simulink model "v2x_cs"  (R2019a)
settings: Solver=ode5  StartTime=0.0  StopTime=inf  FixedStep=1/20  RelTol=1e-3
PreLoadFcn:
  | mbxruntime.callbacks.PreLoadFcn(bdroot);
PostLoadFcn:
  | mbxruntime.callbacks.PostLoadFcn(bdroot);
InitFcn:
  | mbxruntime.callbacks.InitFcn(bdroot);
StartFcn:
  | mbxruntime.callbacks.StartFcn(bdroot);
StopFcn:
  | mbxruntime.callbacks.StopFcn(bdroot);
model workspace (MAT data in the model file):
  mbox_table : struct (value not decoded)
  model_closed = 0
  sim_status = 0
undefined symbols (not defined in the file or in its folder): DiscIntNeverNeededParam, SteeringWheel
libraries: PreScanSimulinkLibrary x10
(part 4 of 5)

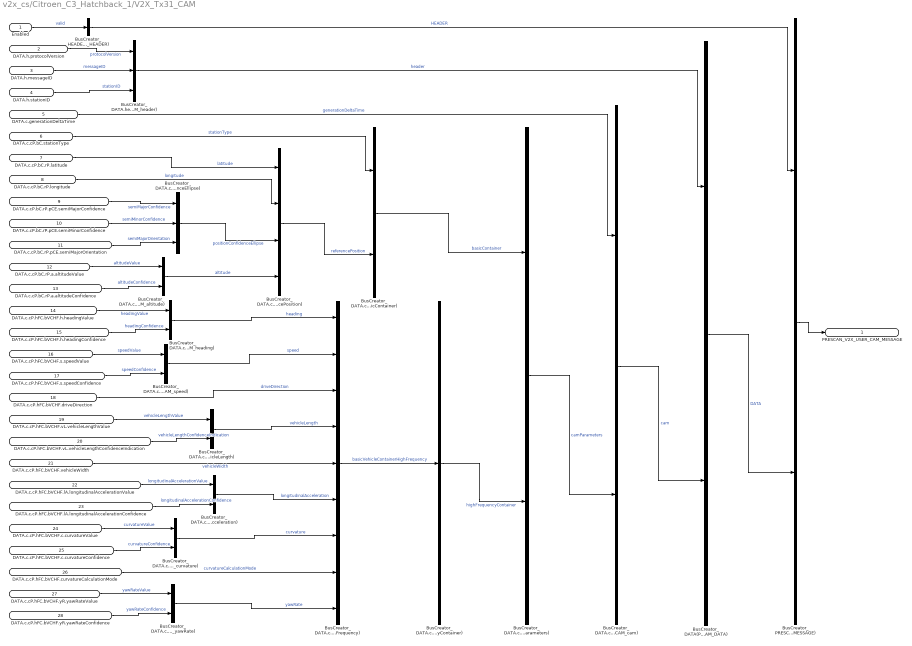
== system v2x_cs/Citroen_C3_Hatchback_1/V2X_Tx31_CAM ==
  Enabled : Inport
  DATA.h.protocolVersion : Inport  Port=2
  DATA.h.messageID : Inport  Port=3
  DATA.h.stationID : Inport  Port=4
  DATA.c.generationDeltaTime : Inport  Port=5
  DATA.c.cP.bC.stationType : Inport  Port=6
  DATA.c.cP.bC.rP.latitude : Inport  Port=7
  DATA.c.cP.bC.rP.longitude : Inport  Port=8
  DATA.c.cP.bC.rP.pCE.semiMajorConfidence : Inport  Port=9
  DATA.c.cP.bC.rP.pCE.semiMinorConfidence : Inport  Port=10
  DATA.c.cP.bC.rP.pCE.semiMajorOrientation : Inport  Port=11
  DATA.c.cP.bC.rP.a.altitudeValue : Inport  Port=12
  DATA.c.cP.bC.rP.a.altitudeConfidence : Inport  Port=13
  DATA.c.cP.hFC.bVCHF.h.headingValue : Inport  Port=14
  DATA.c.cP.hFC.bVCHF.h.headingConfidence : Inport  Port=15
  DATA.c.cP.hFC.bVCHF.s.speedValue : Inport  Port=16
  DATA.c.cP.hFC.bVCHF.s.speedConfidence : Inport  Port=17
  DATA.c.cP.hFC.bVCHF.driveDirection : Inport  Port=18
  DATA.c.cP.hFC.bVCHF.vL.vehicleLengthValue : Inport  Port=19
  DATA.c.cP.hFC.bVCHF.vL.vehicleLengthConfidenceIndication : Inport  Port=20
  DATA.c.cP.hFC.bVCHF.vehicleWidth : Inport  Port=21
  DATA.c.cP.hFC.bVCHF.lA.longitudinalAccelerationValue : Inport  Port=22
  DATA.c.cP.hFC.bVCHF.lA.longitudinalAccelerationConfidence : Inport  Port=23
  DATA.c.cP.hFC.bVCHF.c.curvatureValue : Inport  Port=24
  DATA.c.cP.hFC.bVCHF.c.curvatureConfidence : Inport  Port=25
  DATA.c.cP.hFC.bVCHF.curvatureCalculationMode : Inport  Port=26
  DATA.c.cP.hFC.bVCHF.yR.yawRateValue : Inport  Port=27
  DATA.c.cP.hFC.bVCHF.yR.yawRateConfidence : Inport  Port=28
  BusCreator_DATA(PRESCAN_V2X_USER_CAM_DATA) : BusCreator  Inputs=2  OutDataTypeStr=Bus: PRESCAN_V2X_USER_CAM_DATA  NonVirtualBus=on
  BusCreator_DATA.c.cP.bC.rP.altitude(PRESCAN_V2X_USER_CAM_altitude) : BusCreator  Inputs=2  OutDataTypeStr=Bus: PRESCAN_V2X_USER_CAM_altitude  NonVirtualBus=on
  BusCreator_DATA.c.cP.bC.rP.positionConfidenceEllipse(PRESCAN_V2X_USER_CAM_positionConfidenceEllipse) : BusCreator  Inputs=3  OutDataTypeStr=Bus: PRESCAN_V2X_USER_CAM_positionConfidenceEllipse  NonVirtualBus=on
  BusCreator_DATA.c.cP.bC.referencePosition(PRESCAN_V2X_USER_CAM_referencePosition) : BusCreator  Inputs=4  OutDataTypeStr=Bus: PRESCAN_V2X_USER_CAM_referencePosition  NonVirtualBus=on
  BusCreator_DATA.c.cP.basicContainer(PRESCAN_V2X_USER_CAM_basicContainer) : BusCreator  Inputs=2  OutDataTypeStr=Bus: PRESCAN_V2X_USER_CAM_basicContainer  NonVirtualBus=on
  BusCreator_DATA.c.cP.hFC.bVCHF.curvature(PRESCAN_V2X_USER_CAM_curvature) : BusCreator  Inputs=2  OutDataTypeStr=Bus: PRESCAN_V2X_USER_CAM_curvature  NonVirtualBus=on
  BusCreator_DATA.c.cP.hFC.bVCHF.heading(PRESCAN_V2X_USER_CAM_heading) : BusCreator  Inputs=2  OutDataTypeStr=Bus: PRESCAN_V2X_USER_CAM_heading  NonVirtualBus=on
  BusCreator_DATA.c.cP.hFC.bVCHF.longitudinalAcceleration(PRESCAN_V2X_USER_CAM_longitudinalAcceleration) : BusCreator  Inputs=2  OutDataTypeStr=Bus: PRESCAN_V2X_USER_CAM_longitudinalAcceleration  NonVirtualBus=on
  BusCreator_DATA.c.cP.hFC.bVCHF.speed(PRESCAN_V2X_USER_CAM_speed) : BusCreator  Inputs=2  OutDataTypeStr=Bus: PRESCAN_V2X_USER_CAM_speed  NonVirtualBus=on
  BusCreator_DATA.c.cP.hFC.bVCHF.vehicleLength(PRESCAN_V2X_USER_CAM_vehicleLength) : BusCreator  Inputs=2  OutDataTypeStr=Bus: PRESCAN_V2X_USER_CAM_vehicleLength  NonVirtualBus=on
  BusCreator_DATA.c.cP.hFC.bVCHF.yawRate(PRESCAN_V2X_USER_CAM_yawRate) : BusCreator  Inputs=2  OutDataTypeStr=Bus: PRESCAN_V2X_USER_CAM_yawRate  NonVirtualBus=on
  BusCreator_DATA.c.cP.hFC.basicVehicleContainerHighFrequency(PRESCAN_V2X_USER_CAM_basicVehicleContainerHighFrequency) : BusCreator  Inputs=9  OutDataTypeStr=Bus: PRESCAN_V2X_USER_CAM_basicVehicleContainerHighFrequency  NonVirtualBus=on
  BusCreator_DATA.c.cP.highFrequencyContainer(PRESCAN_V2X_USER_CAM_highFrequencyContainer) : BusCreator  Inputs=1  OutDataTypeStr=Bus: PRESCAN_V2X_USER_CAM_highFrequencyContainer  NonVirtualBus=on
  BusCreator_DATA.c.camParameters(PRESCAN_V2X_USER_CAM_camParameters) : BusCreator  Inputs=2  OutDataTypeStr=Bus: PRESCAN_V2X_USER_CAM_camParameters  NonVirtualBus=on
  BusCreator_DATA.cam(PRESCAN_V2X_USER_CAM_cam) : BusCreator  Inputs=2  OutDataTypeStr=Bus: PRESCAN_V2X_USER_CAM_cam  NonVirtualBus=on
  BusCreator_DATA.header(PRESCAN_V2X_USER_CAM_header) : BusCreator  Inputs=3  OutDataTypeStr=Bus: PRESCAN_V2X_USER_CAM_header  NonVirtualBus=on
  BusCreator_HEADER(PRESCAN_HEADER) : BusCreator  Inputs=1  OutDataTypeStr=Bus: PRESCAN_HEADER  NonVirtualBus=on
  BusCreator_PRESCAN_V2X_USER_CAM_MESSAGE(PRESCAN_V2X_USER_CAM_MESSAGE) : BusCreator  Inputs=2  OutDataTypeStr=Bus: PRESCAN_V2X_USER_CAM_MESSAGE  NonVirtualBus=on
  PRESCAN_V2X_USER_CAM_MESSAGE : Outport
  wires:
  Enabled/1 -> BusCreator_HEADER(PRESCAN_HEADER)/1  "valid"
  DATA.h.messageID/1 -> BusCreator_DATA.header(PRESCAN_V2X_USER_CAM_header)/2  "messageID"
  DATA.h.stationID/1 -> BusCreator_DATA.header(PRESCAN_V2X_USER_CAM_header)/3  "stationID"
  DATA.h.protocolVersion/1 -> BusCreator_DATA.header(PRESCAN_V2X_USER_CAM_header)/1  "protocolVersion"
  DATA.c.cP.bC.rP.pCE.semiMinorConfidence/1 -> BusCreator_DATA.c.cP.bC.rP.positionConfidenceEllipse(PRESCAN_V2X_USER_CAM_positionConfidenceEllipse)/2  "semiMinorConfidence"
  DATA.c.cP.bC.rP.pCE.semiMajorOrientation/1 -> BusCreator_DATA.c.cP.bC.rP.positionConfidenceEllipse(PRESCAN_V2X_USER_CAM_positionConfidenceEllipse)/3  "semiMajorOrientation"
  DATA.c.cP.bC.rP.pCE.semiMajorConfidence/1 -> BusCreator_DATA.c.cP.bC.rP.positionConfidenceEllipse(PRESCAN_V2X_USER_CAM_positionConfidenceEllipse)/1  "semiMajorConfidence"
  DATA.c.cP.bC.rP.a.altitudeValue/1 -> BusCreator_DATA.c.cP.bC.rP.altitude(PRESCAN_V2X_USER_CAM_altitude)/1  "altitudeValue"
  DATA.c.cP.bC.rP.a.altitudeConfidence/1 -> BusCreator_DATA.c.cP.bC.rP.altitude(PRESCAN_V2X_USER_CAM_altitude)/2  "altitudeConfidence"
  DATA.c.cP.bC.rP.longitude/1 -> BusCreator_DATA.c.cP.bC.referencePosition(PRESCAN_V2X_USER_CAM_referencePosition)/2  "longitude"
  BusCreator_DATA.c.cP.bC.rP.positionConfidenceEllipse(PRESCAN_V2X_USER_CAM_positionConfidenceEllipse)/1 -> BusCreator_DATA.c.cP.bC.referencePosition(PRESCAN_V2X_USER_CAM_referencePosition)/3  "positionConfidenceEllipse"
  DATA.c.cP.bC.rP.latitude/1 -> BusCreator_DATA.c.cP.bC.referencePosition(PRESCAN_V2X_USER_CAM_referencePosition)/1  "latitude"
  BusCreator_DATA.c.cP.bC.rP.altitude(PRESCAN_V2X_USER_CAM_altitude)/1 -> BusCreator_DATA.c.cP.bC.referencePosition(PRESCAN_V2X_USER_CAM_referencePosition)/4  "altitude"
  DATA.c.cP.bC.stationType/1 -> BusCreator_DATA.c.cP.basicContainer(PRESCAN_V2X_USER_CAM_basicContainer)/1  "stationType"
  BusCreator_DATA.c.cP.bC.referencePosition(PRESCAN_V2X_USER_CAM_referencePosition)/1 -> BusCreator_DATA.c.cP.basicContainer(PRESCAN_V2X_USER_CAM_basicContainer)/2  "referencePosition"
  DATA.c.cP.hFC.bVCHF.h.headingValue/1 -> BusCreator_DATA.c.cP.hFC.bVCHF.heading(PRESCAN_V2X_USER_CAM_heading)/1  "headingValue"
  DATA.c.cP.hFC.bVCHF.h.headingConfidence/1 -> BusCreator_DATA.c.cP.hFC.bVCHF.heading(PRESCAN_V2X_USER_CAM_heading)/2  "headingConfidence"
  DATA.c.cP.hFC.bVCHF.s.speedValue/1 -> BusCreator_DATA.c.cP.hFC.bVCHF.speed(PRESCAN_V2X_USER_CAM_speed)/1  "speedValue"
  DATA.c.cP.hFC.bVCHF.s.speedConfidence/1 -> BusCreator_DATA.c.cP.hFC.bVCHF.speed(PRESCAN_V2X_USER_CAM_speed)/2  "speedConfidence"
  DATA.c.cP.hFC.bVCHF.vL.vehicleLengthValue/1 -> BusCreator_DATA.c.cP.hFC.bVCHF.vehicleLength(PRESCAN_V2X_USER_CAM_vehicleLength)/1  "vehicleLengthValue"
  DATA.c.cP.hFC.bVCHF.vL.vehicleLengthConfidenceIndication/1 -> BusCreator_DATA.c.cP.hFC.bVCHF.vehicleLength(PRESCAN_V2X_USER_CAM_vehicleLength)/2  "vehicleLengthConfidenceIndication"
  DATA.c.cP.hFC.bVCHF.lA.longitudinalAccelerationValue/1 -> BusCreator_DATA.c.cP.hFC.bVCHF.longitudinalAcceleration(PRESCAN_V2X_USER_CAM_longitudinalAcceleration)/1  "longitudinalAccelerationValue"
  DATA.c.cP.hFC.bVCHF.lA.longitudinalAccelerationConfidence/1 -> BusCreator_DATA.c.cP.hFC.bVCHF.longitudinalAcceleration(PRESCAN_V2X_USER_CAM_longitudinalAcceleration)/2  "longitudinalAccelerationConfidence"
  DATA.c.cP.hFC.bVCHF.c.curvatureValue/1 -> BusCreator_DATA.c.cP.hFC.bVCHF.curvature(PRESCAN_V2X_USER_CAM_curvature)/1  "curvatureValue"
  DATA.c.cP.hFC.bVCHF.c.curvatureConfidence/1 -> BusCreator_DATA.c.cP.hFC.bVCHF.curvature(PRESCAN_V2X_USER_CAM_curvature)/2  "curvatureConfidence"
  DATA.c.cP.hFC.bVCHF.yR.yawRateValue/1 -> BusCreator_DATA.c.cP.hFC.bVCHF.yawRate(PRESCAN_V2X_USER_CAM_yawRate)/1  "yawRateValue"
  DATA.c.cP.hFC.bVCHF.yR.yawRateConfidence/1 -> BusCreator_DATA.c.cP.hFC.bVCHF.yawRate(PRESCAN_V2X_USER_CAM_yawRate)/2  "yawRateConfidence"
  DATA.c.cP.hFC.bVCHF.vehicleWidth/1 -> BusCreator_DATA.c.cP.hFC.basicVehicleContainerHighFrequency(PRESCAN_V2X_USER_CAM_basicVehicleContainerHighFrequency)/5  "vehicleWidth"
  BusCreator_DATA.c.cP.hFC.bVCHF.longitudinalAcceleration(PRESCAN_V2X_USER_CAM_longitudinalAcceleration)/1 -> BusCreator_DATA.c.cP.hFC.basicVehicleContainerHighFrequency(PRESCAN_V2X_USER_CAM_basicVehicleContainerHighFrequency)/6  "longitudinalAcceleration"
  BusCreator_DATA.c.cP.hFC.bVCHF.vehicleLength(PRESCAN_V2X_USER_CAM_vehicleLength)/1 -> BusCreator_DATA.c.cP.hFC.basicVehicleContainerHighFrequency(PRESCAN_V2X_USER_CAM_basicVehicleContainerHighFrequency)/4  "vehicleLength"
  BusCreator_DATA.c.cP.hFC.bVCHF.curvature(PRESCAN_V2X_USER_CAM_curvature)/1 -> BusCreator_DATA.c.cP.hFC.basicVehicleContainerHighFrequency(PRESCAN_V2X_USER_CAM_basicVehicleContainerHighFrequency)/7  "curvature"
  DATA.c.cP.hFC.bVCHF.driveDirection/1 -> BusCreator_DATA.c.cP.hFC.basicVehicleContainerHighFrequency(PRESCAN_V2X_USER_CAM_basicVehicleContainerHighFrequency)/3  "driveDirection"
  DATA.c.cP.hFC.bVCHF.curvatureCalculationMode/1 -> BusCreator_DATA.c.cP.hFC.basicVehicleContainerHighFrequency(PRESCAN_V2X_USER_CAM_basicVehicleContainerHighFrequency)/8  "curvatureCalculationMode"
  BusCreator_DATA.c.cP.hFC.bVCHF.speed(PRESCAN_V2X_USER_CAM_speed)/1 -> BusCreator_DATA.c.cP.hFC.basicVehicleContainerHighFrequency(PRESCAN_V2X_USER_CAM_basicVehicleContainerHighFrequency)/2  "speed"
  BusCreator_DATA.c.cP.hFC.bVCHF.yawRate(PRESCAN_V2X_USER_CAM_yawRate)/1 -> BusCreator_DATA.c.cP.hFC.basicVehicleContainerHighFrequency(PRESCAN_V2X_USER_CAM_basicVehicleContainerHighFrequency)/9  "yawRate"
  BusCreator_DATA.c.cP.hFC.bVCHF.heading(PRESCAN_V2X_USER_CAM_heading)/1 -> BusCreator_DATA.c.cP.hFC.basicVehicleContainerHighFrequency(PRESCAN_V2X_USER_CAM_basicVehicleContainerHighFrequency)/1  "heading"
  BusCreator_DATA.c.cP.hFC.basicVehicleContainerHighFrequency(PRESCAN_V2X_USER_CAM_basicVehicleContainerHighFrequency)/1 -> BusCreator_DATA.c.cP.highFrequencyContainer(PRESCAN_V2X_USER_CAM_highFrequencyContainer)/1  "basicVehicleContainerHighFrequency"
  BusCreator_DATA.c.cP.basicContainer(PRESCAN_V2X_USER_CAM_basicContainer)/1 -> BusCreator_DATA.c.camParameters(PRESCAN_V2X_USER_CAM_camParameters)/1  "basicContainer"
  BusCreator_DATA.c.cP.highFrequencyContainer(PRESCAN_V2X_USER_CAM_highFrequencyContainer)/1 -> BusCreator_DATA.c.camParameters(PRESCAN_V2X_USER_CAM_camParameters)/2  "highFrequencyContainer"
  DATA.c.generationDeltaTime/1 -> BusCreator_DATA.cam(PRESCAN_V2X_USER_CAM_cam)/1  "generationDeltaTime"
  BusCreator_DATA.c.camParameters(PRESCAN_V2X_USER_CAM_camParameters)/1 -> BusCreator_DATA.cam(PRESCAN_V2X_USER_CAM_cam)/2  "camParameters"
  BusCreator_DATA.header(PRESCAN_V2X_USER_CAM_header)/1 -> BusCreator_DATA(PRESCAN_V2X_USER_CAM_DATA)/1  "header"
  BusCreator_DATA.cam(PRESCAN_V2X_USER_CAM_cam)/1 -> BusCreator_DATA(PRESCAN_V2X_USER_CAM_DATA)/2  "cam"
  BusCreator_HEADER(PRESCAN_HEADER)/1 -> BusCreator_PRESCAN_V2X_USER_CAM_MESSAGE(PRESCAN_V2X_USER_CAM_MESSAGE)/1  "HEADER"
  BusCreator_DATA(PRESCAN_V2X_USER_CAM_DATA)/1 -> BusCreator_PRESCAN_V2X_USER_CAM_MESSAGE(PRESCAN_V2X_USER_CAM_MESSAGE)/2  "DATA"
  BusCreator_PRESCAN_V2X_USER_CAM_MESSAGE(PRESCAN_V2X_USER_CAM_MESSAGE)/1 -> PRESCAN_V2X_USER_CAM_MESSAGE/1

== system v2x_cs/Mazda_RX8_Coupe_1/Dynamics_Empty ==
  note: For state mode 'Dynamic' positions
      | are not taken into account, as they
      | are computed by integrating velocity.
      | Click annotation for Help.
  Ground_{1..9} (9 alike) : Ground
  MuxState : Subsystem  Tag=mux/State  mask(Empty Dynamics State Block){positioningmode=on, TimeStep=1/20}
      mask prompts: positioningmode "Positioning Mode"; TimeStep "Auto Assigned: Time Step [s]"
      mask help:
      | Build the state of an actor based on user input.
      | The user can either use positioning mode or dynamics mode.
      | - When using positioning mode the position and orientation of the actor are set directly based on the input. Expected input is relative to the initial position and orientation of the actor. It's also possible to specify the velocity of the actor, though this input isn't used, only passed on.
      | - When using dynamics mode the position input is ignored. Expected input is velocity and orientation. The velocity is relative the current orientation of the actor, while orientation is relative to its initial orientation. The position of the actor is calculated based on the velocity and orientation given.
      settings: DeleteFcn=PreScanBlockDeleteFcn;
  State : Outport  Tag=outport/StateOutport  SampleTime=1/20
  wires:
  MuxState/1(state) -> State/1
  Ground_1/1 -> MuxState/1(x [m])
  Ground_2/1 -> MuxState/2(y [m])
  Ground_3/1 -> MuxState/3(z [m])
  Ground_4/1 -> MuxState/4(dx [m/s])
  Ground_5/1 -> MuxState/5(dy [m/s])
  Ground_6/1 -> MuxState/6(dz [m/s])
  Ground_7/1 -> MuxState/7(R [rad])
  Ground_8/1 -> MuxState/8(P [rad])
  Ground_9/1 -> MuxState/9(Y [rad])

== system v2x_cs/Mazda_RX8_Coupe_1/SELF_Demux ==
  SELF : Inport  OutDataTypeStr=Bus: PRESCAN_SELFSENSORDATA
  Bus Selector : BusSelector  OutputSignals=PositionX,PositionY,PositionZ,OrientationRoll,OrientationPitch,OrientationYaw,Velocity,Yaw_rate,Lat,Long,Alt
  Demux2 : Demux  Outputs=3
  Gain : Gain  Gain=180/pi
  Gain1 : Gain  Gain=180/pi
  Vector Concatenate1 : Concatenate  NumInputs=3
  compas converter : Subsystem
  x [m] : Outport
  y [m] : Outport  Port=2
  z [m] : Outport  Port=3
  rotx [deg] : Outport  Port=4
  roty [deg] : Outport  Port=5
  rotz [deg] : Outport  Port=6
  GPS lat [deg] : Outport  Port=7
  GPS long [deg] : Outport  Port=8
  GPS alt [m] : Outport  Port=9
  velocity [m/s] : Outport  Port=10
  heading [deg] : Outport  Port=11
  yaw rate [deg/s] : Outport  Port=12
  wires:
  Bus Selector/11 -> GPS alt [m]/1  "<Alt>"
  Bus Selector/10 -> GPS long [deg]/1  "<Long>"
  Bus Selector/9 -> GPS lat [deg]/1  "<Lat>"
  Bus Selector/8 -> Gain1/1  "<Yaw_rate>"
  Bus Selector/7 -> velocity [m/s]/1  "<Velocity>"
  Bus Selector/6 -> compas converter/1(rotz [rad]), Vector Concatenate1/3  "<OrientationYaw>"
  Bus Selector/5 -> Vector Concatenate1/2  "<OrientationPitch>"
  Bus Selector/4 -> Vector Concatenate1/1  "<OrientationRoll>"
  Vector Concatenate1/1 -> Gain/1
  Bus Selector/3 -> z [m]/1  "<PositionZ>"
  Bus Selector/2 -> y [m]/1  "<PositionY>"
  Bus Selector/1 -> x [m]/1  "<PositionX>"
  SELF/1 -> Bus Selector/1
  Gain/1 -> Demux2/1
  Demux2/1 -> rotx [deg]/1
  Demux2/2 -> roty [deg]/1
  Demux2/3 -> rotz [deg]/1
  compas converter/1(heading [deg]) -> heading [deg]/1
  Gain1/1 -> yaw rate [deg/s]/1

== system v2x_cs/Mazda_RX8_Coupe_1/STATE_Mazda_RX8_Coupe_1 ==
  State : Inport  SampleTime=TimeStep
  Bus Creator : BusCreator  Inputs=15  OutDataTypeStr=Bus: PRESCAN_STATEACTUATORDATA  NonVirtualBus=on
  Demux : Demux  Outputs=15
  iniBODYAngles wrtVEH [rad] : Constant  Value=[Roll0 Pitch0 0]  SampleTime=TimeStep
  iniVEHAngles wrtGLOB [rad] : Constant  Value=[0 0 Yaw0]  SampleTime=TimeStep
  iniVEHposition wrtGLOB [m] : Constant  Value=[x0 y0 z0]  SampleTime=TimeStep
  state2FullState : PreScanSimulinkLibrary/state2FullState  SystemSampleTime=-1
  StateBus : Outport  OutDataTypeStr=Bus: PRESCAN_STATEACTUATORDATA
  wires:
  Bus Creator/1 -> StateBus/1
  State/1 -> state2FullState/1
  state2FullState/1 -> Demux/1
  iniVEHposition wrtGLOB [m]/1 -> state2FullState/2
  iniBODYAngles wrtVEH [rad]/1 -> state2FullState/3
  iniVEHAngles wrtGLOB [rad]/1 -> state2FullState/4
  Demux/1 -> Bus Creator/1  "PositionX"
  Demux/2 -> Bus Creator/2  "PositionY"
  Demux/3 -> Bus Creator/3  "PositionZ"
  Demux/4 -> Bus Creator/4  "VelocityX"
  Demux/5 -> Bus Creator/5  "VelocityY"
  Demux/6 -> Bus Creator/6  "VelocityZ"
  Demux/7 -> Bus Creator/7  "AccelerationX"
  Demux/8 -> Bus Creator/8  "AccelerationY"
  Demux/9 -> Bus Creator/9  "AccelerationZ"
  Demux/10 -> Bus Creator/10  "OrientationRoll"
  Demux/11 -> Bus Creator/11  "OrientationPitch"
  Demux/12 -> Bus Creator/12  "OrientationYaw"
  Demux/13 -> Bus Creator/13  "AngularVelocityRoll"
  Demux/14 -> Bus Creator/14  "AngularVelocityPitch"
  Demux/15 -> Bus Creator/15  "AngularVelocityYaw"

== system v2x_cs/Mazda_RX8_Coupe_1/SteeringWheel_pivot_Mux ==
  X [m] : Inport
  Y [m] : Inport  Port=2
  Z [m] : Inport  Port=3
  Roll [rad] : Inport  Port=4
  Pitch [rad] : Inport  Port=5
  Yaw [rad] : Inport  Port=6
  Bus Creator : BusCreator  Inputs=3  OutDataTypeStr=Bus: PRESCAN_XYZ_DATA
  Bus Creator1 : BusCreator  Inputs=3  OutDataTypeStr=Bus: PRESCAN_RPY_DATA
  Bus Creator2 : BusCreator  Inputs=2  OutDataTypeStr=Bus: PRESCAN_POSE_DATA
  Joint : Outport
  wires:
  Yaw [rad]/1 -> Bus Creator1/3  "Yaw"
  Bus Creator1/1 -> Bus Creator2/2  "ORIENTATION"
  Bus Creator/1 -> Bus Creator2/1  "POSITION"
  X [m]/1 -> Bus Creator/1  "X"
  Y [m]/1 -> Bus Creator/2  "Y"
  Z [m]/1 -> Bus Creator/3  "Z"
  Bus Creator2/1 -> Joint/1
  Roll [rad]/1 -> Bus Creator1/1  "Roll"
  Pitch [rad]/1 -> Bus Creator1/2  "Pitch"

== system v2x_cs/Mazda_RX8_Coupe_1/V2X_27_CAM_Expander ==
  In : Inport
  Expander : MATLAB Function  TreatAsAtomicUnit=on
  Zero : Constant  Value=0  OutDataTypeStr=Bus: PRESCAN_V2X_FIXED_CAM_MESSAGE
  Out : Outport
  wires:
  In/1 -> Expander/1(u)
  Expander/1(y) -> Out/1
  Zero/1 -> Expander/2(z)

== system v2x_cs/Mazda_RX8_Coupe_1/V2X_27_CAM_Filter ==
  Filter_In : Inport  Partition=on  PartitionDimension=1  PartitionWidth=1  PartitionOffset=0
  Filter : Subsystem
  ForEach : ForEach
  Filter_Out : Outport  ConcatenationDimension=1
  wires:
  Filter_In/1 -> Filter/1(In)
  Filter/1(Out) -> Filter_Out/1

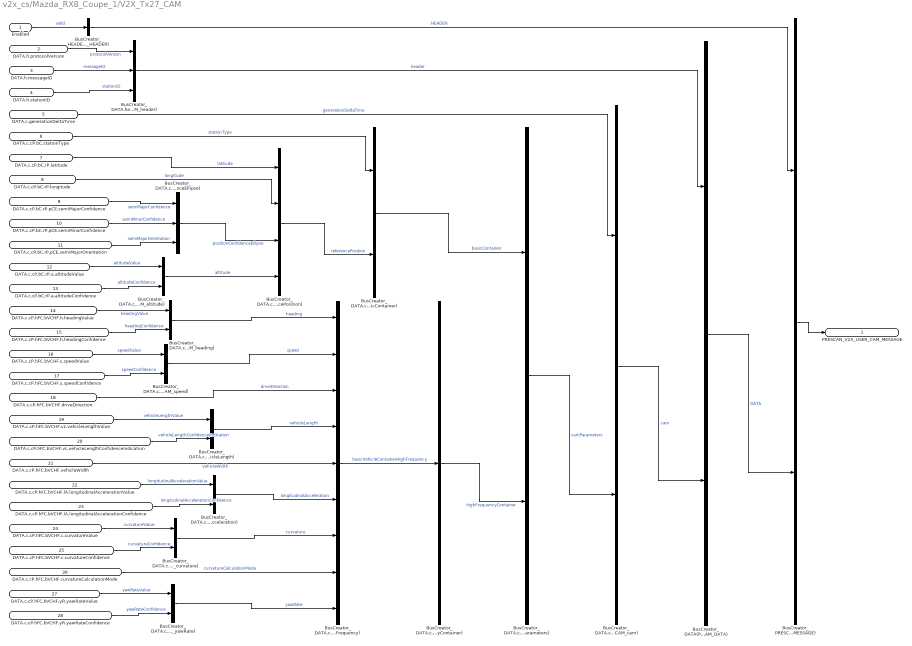
== system v2x_cs/Mazda_RX8_Coupe_1/V2X_Tx27_CAM ==
  Enabled : Inport
  DATA.h.protocolVersion : Inport  Port=2
  DATA.h.messageID : Inport  Port=3
  DATA.h.stationID : Inport  Port=4
  DATA.c.generationDeltaTime : Inport  Port=5
  DATA.c.cP.bC.stationType : Inport  Port=6
  DATA.c.cP.bC.rP.latitude : Inport  Port=7
  DATA.c.cP.bC.rP.longitude : Inport  Port=8
  DATA.c.cP.bC.rP.pCE.semiMajorConfidence : Inport  Port=9
  DATA.c.cP.bC.rP.pCE.semiMinorConfidence : Inport  Port=10
  DATA.c.cP.bC.rP.pCE.semiMajorOrientation : Inport  Port=11
  DATA.c.cP.bC.rP.a.altitudeValue : Inport  Port=12
  DATA.c.cP.bC.rP.a.altitudeConfidence : Inport  Port=13
  DATA.c.cP.hFC.bVCHF.h.headingValue : Inport  Port=14
  DATA.c.cP.hFC.bVCHF.h.headingConfidence : Inport  Port=15
  DATA.c.cP.hFC.bVCHF.s.speedValue : Inport  Port=16
  DATA.c.cP.hFC.bVCHF.s.speedConfidence : Inport  Port=17
  DATA.c.cP.hFC.bVCHF.driveDirection : Inport  Port=18
  DATA.c.cP.hFC.bVCHF.vL.vehicleLengthValue : Inport  Port=19
  DATA.c.cP.hFC.bVCHF.vL.vehicleLengthConfidenceIndication : Inport  Port=20
  DATA.c.cP.hFC.bVCHF.vehicleWidth : Inport  Port=21
  DATA.c.cP.hFC.bVCHF.lA.longitudinalAccelerationValue : Inport  Port=22
  DATA.c.cP.hFC.bVCHF.lA.longitudinalAccelerationConfidence : Inport  Port=23
  DATA.c.cP.hFC.bVCHF.c.curvatureValue : Inport  Port=24
  DATA.c.cP.hFC.bVCHF.c.curvatureConfidence : Inport  Port=25
  DATA.c.cP.hFC.bVCHF.curvatureCalculationMode : Inport  Port=26
  DATA.c.cP.hFC.bVCHF.yR.yawRateValue : Inport  Port=27
  DATA.c.cP.hFC.bVCHF.yR.yawRateConfidence : Inport  Port=28
  BusCreator_DATA(PRESCAN_V2X_USER_CAM_DATA) : BusCreator  Inputs=2  OutDataTypeStr=Bus: PRESCAN_V2X_USER_CAM_DATA  NonVirtualBus=on
  BusCreator_DATA.c.cP.bC.rP.altitude(PRESCAN_V2X_USER_CAM_altitude) : BusCreator  Inputs=2  OutDataTypeStr=Bus: PRESCAN_V2X_USER_CAM_altitude  NonVirtualBus=on
  BusCreator_DATA.c.cP.bC.rP.positionConfidenceEllipse(PRESCAN_V2X_USER_CAM_positionConfidenceEllipse) : BusCreator  Inputs=3  OutDataTypeStr=Bus: PRESCAN_V2X_USER_CAM_positionConfidenceEllipse  NonVirtualBus=on
  BusCreator_DATA.c.cP.bC.referencePosition(PRESCAN_V2X_USER_CAM_referencePosition) : BusCreator  Inputs=4  OutDataTypeStr=Bus: PRESCAN_V2X_USER_CAM_referencePosition  NonVirtualBus=on
  BusCreator_DATA.c.cP.basicContainer(PRESCAN_V2X_USER_CAM_basicContainer) : BusCreator  Inputs=2  OutDataTypeStr=Bus: PRESCAN_V2X_USER_CAM_basicContainer  NonVirtualBus=on
  BusCreator_DATA.c.cP.hFC.bVCHF.curvature(PRESCAN_V2X_USER_CAM_curvature) : BusCreator  Inputs=2  OutDataTypeStr=Bus: PRESCAN_V2X_USER_CAM_curvature  NonVirtualBus=on
  BusCreator_DATA.c.cP.hFC.bVCHF.heading(PRESCAN_V2X_USER_CAM_heading) : BusCreator  Inputs=2  OutDataTypeStr=Bus: PRESCAN_V2X_USER_CAM_heading  NonVirtualBus=on
  BusCreator_DATA.c.cP.hFC.bVCHF.longitudinalAcceleration(PRESCAN_V2X_USER_CAM_longitudinalAcceleration) : BusCreator  Inputs=2  OutDataTypeStr=Bus: PRESCAN_V2X_USER_CAM_longitudinalAcceleration  NonVirtualBus=on
  BusCreator_DATA.c.cP.hFC.bVCHF.speed(PRESCAN_V2X_USER_CAM_speed) : BusCreator  Inputs=2  OutDataTypeStr=Bus: PRESCAN_V2X_USER_CAM_speed  NonVirtualBus=on
  BusCreator_DATA.c.cP.hFC.bVCHF.vehicleLength(PRESCAN_V2X_USER_CAM_vehicleLength) : BusCreator  Inputs=2  OutDataTypeStr=Bus: PRESCAN_V2X_USER_CAM_vehicleLength  NonVirtualBus=on
  BusCreator_DATA.c.cP.hFC.bVCHF.yawRate(PRESCAN_V2X_USER_CAM_yawRate) : BusCreator  Inputs=2  OutDataTypeStr=Bus: PRESCAN_V2X_USER_CAM_yawRate  NonVirtualBus=on
  BusCreator_DATA.c.cP.hFC.basicVehicleContainerHighFrequency(PRESCAN_V2X_USER_CAM_basicVehicleContainerHighFrequency) : BusCreator  Inputs=9  OutDataTypeStr=Bus: PRESCAN_V2X_USER_CAM_basicVehicleContainerHighFrequency  NonVirtualBus=on
  BusCreator_DATA.c.cP.highFrequencyContainer(PRESCAN_V2X_USER_CAM_highFrequencyContainer) : BusCreator  Inputs=1  OutDataTypeStr=Bus: PRESCAN_V2X_USER_CAM_highFrequencyContainer  NonVirtualBus=on
  BusCreator_DATA.c.camParameters(PRESCAN_V2X_USER_CAM_camParameters) : BusCreator  Inputs=2  OutDataTypeStr=Bus: PRESCAN_V2X_USER_CAM_camParameters  NonVirtualBus=on
  BusCreator_DATA.cam(PRESCAN_V2X_USER_CAM_cam) : BusCreator  Inputs=2  OutDataTypeStr=Bus: PRESCAN_V2X_USER_CAM_cam  NonVirtualBus=on
  BusCreator_DATA.header(PRESCAN_V2X_USER_CAM_header) : BusCreator  Inputs=3  OutDataTypeStr=Bus: PRESCAN_V2X_USER_CAM_header  NonVirtualBus=on
  BusCreator_HEADER(PRESCAN_HEADER) : BusCreator  Inputs=1  OutDataTypeStr=Bus: PRESCAN_HEADER  NonVirtualBus=on
  BusCreator_PRESCAN_V2X_USER_CAM_MESSAGE(PRESCAN_V2X_USER_CAM_MESSAGE) : BusCreator  Inputs=2  OutDataTypeStr=Bus: PRESCAN_V2X_USER_CAM_MESSAGE  NonVirtualBus=on
  PRESCAN_V2X_USER_CAM_MESSAGE : Outport
  wires:
  Enabled/1 -> BusCreator_HEADER(PRESCAN_HEADER)/1  "valid"
  DATA.h.messageID/1 -> BusCreator_DATA.header(PRESCAN_V2X_USER_CAM_header)/2  "messageID"
  DATA.h.stationID/1 -> BusCreator_DATA.header(PRESCAN_V2X_USER_CAM_header)/3  "stationID"
  DATA.h.protocolVersion/1 -> BusCreator_DATA.header(PRESCAN_V2X_USER_CAM_header)/1  "protocolVersion"
  DATA.c.cP.bC.rP.pCE.semiMinorConfidence/1 -> BusCreator_DATA.c.cP.bC.rP.positionConfidenceEllipse(PRESCAN_V2X_USER_CAM_positionConfidenceEllipse)/2  "semiMinorConfidence"
  DATA.c.cP.bC.rP.pCE.semiMajorOrientation/1 -> BusCreator_DATA.c.cP.bC.rP.positionConfidenceEllipse(PRESCAN_V2X_USER_CAM_positionConfidenceEllipse)/3  "semiMajorOrientation"
  DATA.c.cP.bC.rP.pCE.semiMajorConfidence/1 -> BusCreator_DATA.c.cP.bC.rP.positionConfidenceEllipse(PRESCAN_V2X_USER_CAM_positionConfidenceEllipse)/1  "semiMajorConfidence"
  DATA.c.cP.bC.rP.a.altitudeValue/1 -> BusCreator_DATA.c.cP.bC.rP.altitude(PRESCAN_V2X_USER_CAM_altitude)/1  "altitudeValue"
  DATA.c.cP.bC.rP.a.altitudeConfidence/1 -> BusCreator_DATA.c.cP.bC.rP.altitude(PRESCAN_V2X_USER_CAM_altitude)/2  "altitudeConfidence"
  DATA.c.cP.bC.rP.longitude/1 -> BusCreator_DATA.c.cP.bC.referencePosition(PRESCAN_V2X_USER_CAM_referencePosition)/2  "longitude"
  BusCreator_DATA.c.cP.bC.rP.positionConfidenceEllipse(PRESCAN_V2X_USER_CAM_positionConfidenceEllipse)/1 -> BusCreator_DATA.c.cP.bC.referencePosition(PRESCAN_V2X_USER_CAM_referencePosition)/3  "positionConfidenceEllipse"
  DATA.c.cP.bC.rP.latitude/1 -> BusCreator_DATA.c.cP.bC.referencePosition(PRESCAN_V2X_USER_CAM_referencePosition)/1  "latitude"
  BusCreator_DATA.c.cP.bC.rP.altitude(PRESCAN_V2X_USER_CAM_altitude)/1 -> BusCreator_DATA.c.cP.bC.referencePosition(PRESCAN_V2X_USER_CAM_referencePosition)/4  "altitude"
  DATA.c.cP.bC.stationType/1 -> BusCreator_DATA.c.cP.basicContainer(PRESCAN_V2X_USER_CAM_basicContainer)/1  "stationType"
  BusCreator_DATA.c.cP.bC.referencePosition(PRESCAN_V2X_USER_CAM_referencePosition)/1 -> BusCreator_DATA.c.cP.basicContainer(PRESCAN_V2X_USER_CAM_basicContainer)/2  "referencePosition"
  DATA.c.cP.hFC.bVCHF.h.headingValue/1 -> BusCreator_DATA.c.cP.hFC.bVCHF.heading(PRESCAN_V2X_USER_CAM_heading)/1  "headingValue"
  DATA.c.cP.hFC.bVCHF.h.headingConfidence/1 -> BusCreator_DATA.c.cP.hFC.bVCHF.heading(PRESCAN_V2X_USER_CAM_heading)/2  "headingConfidence"
  DATA.c.cP.hFC.bVCHF.s.speedValue/1 -> BusCreator_DATA.c.cP.hFC.bVCHF.speed(PRESCAN_V2X_USER_CAM_speed)/1  "speedValue"
  DATA.c.cP.hFC.bVCHF.s.speedConfidence/1 -> BusCreator_DATA.c.cP.hFC.bVCHF.speed(PRESCAN_V2X_USER_CAM_speed)/2  "speedConfidence"
  DATA.c.cP.hFC.bVCHF.vL.vehicleLengthValue/1 -> BusCreator_DATA.c.cP.hFC.bVCHF.vehicleLength(PRESCAN_V2X_USER_CAM_vehicleLength)/1  "vehicleLengthValue"
  DATA.c.cP.hFC.bVCHF.vL.vehicleLengthConfidenceIndication/1 -> BusCreator_DATA.c.cP.hFC.bVCHF.vehicleLength(PRESCAN_V2X_USER_CAM_vehicleLength)/2  "vehicleLengthConfidenceIndication"
  DATA.c.cP.hFC.bVCHF.lA.longitudinalAccelerationValue/1 -> BusCreator_DATA.c.cP.hFC.bVCHF.longitudinalAcceleration(PRESCAN_V2X_USER_CAM_longitudinalAcceleration)/1  "longitudinalAccelerationValue"
  DATA.c.cP.hFC.bVCHF.lA.longitudinalAccelerationConfidence/1 -> BusCreator_DATA.c.cP.hFC.bVCHF.longitudinalAcceleration(PRESCAN_V2X_USER_CAM_longitudinalAcceleration)/2  "longitudinalAccelerationConfidence"
  DATA.c.cP.hFC.bVCHF.c.curvatureValue/1 -> BusCreator_DATA.c.cP.hFC.bVCHF.curvature(PRESCAN_V2X_USER_CAM_curvature)/1  "curvatureValue"
  DATA.c.cP.hFC.bVCHF.c.curvatureConfidence/1 -> BusCreator_DATA.c.cP.hFC.bVCHF.curvature(PRESCAN_V2X_USER_CAM_curvature)/2  "curvatureConfidence"
  DATA.c.cP.hFC.bVCHF.yR.yawRateValue/1 -> BusCreator_DATA.c.cP.hFC.bVCHF.yawRate(PRESCAN_V2X_USER_CAM_yawRate)/1  "yawRateValue"
  DATA.c.cP.hFC.bVCHF.yR.yawRateConfidence/1 -> BusCreator_DATA.c.cP.hFC.bVCHF.yawRate(PRESCAN_V2X_USER_CAM_yawRate)/2  "yawRateConfidence"
  DATA.c.cP.hFC.bVCHF.vehicleWidth/1 -> BusCreator_DATA.c.cP.hFC.basicVehicleContainerHighFrequency(PRESCAN_V2X_USER_CAM_basicVehicleContainerHighFrequency)/5  "vehicleWidth"
  BusCreator_DATA.c.cP.hFC.bVCHF.longitudinalAcceleration(PRESCAN_V2X_USER_CAM_longitudinalAcceleration)/1 -> BusCreator_DATA.c.cP.hFC.basicVehicleContainerHighFrequency(PRESCAN_V2X_USER_CAM_basicVehicleContainerHighFrequency)/6  "longitudinalAcceleration"
  BusCreator_DATA.c.cP.hFC.bVCHF.vehicleLength(PRESCAN_V2X_USER_CAM_vehicleLength)/1 -> BusCreator_DATA.c.cP.hFC.basicVehicleContainerHighFrequency(PRESCAN_V2X_USER_CAM_basicVehicleContainerHighFrequency)/4  "vehicleLength"
  BusCreator_DATA.c.cP.hFC.bVCHF.curvature(PRESCAN_V2X_USER_CAM_curvature)/1 -> BusCreator_DATA.c.cP.hFC.basicVehicleContainerHighFrequency(PRESCAN_V2X_USER_CAM_basicVehicleContainerHighFrequency)/7  "curvature"
  DATA.c.cP.hFC.bVCHF.driveDirection/1 -> BusCreator_DATA.c.cP.hFC.basicVehicleContainerHighFrequency(PRESCAN_V2X_USER_CAM_basicVehicleContainerHighFrequency)/3  "driveDirection"
  DATA.c.cP.hFC.bVCHF.curvatureCalculationMode/1 -> BusCreator_DATA.c.cP.hFC.basicVehicleContainerHighFrequency(PRESCAN_V2X_USER_CAM_basicVehicleContainerHighFrequency)/8  "curvatureCalculationMode"
  BusCreator_DATA.c.cP.hFC.bVCHF.speed(PRESCAN_V2X_USER_CAM_speed)/1 -> BusCreator_DATA.c.cP.hFC.basicVehicleContainerHighFrequency(PRESCAN_V2X_USER_CAM_basicVehicleContainerHighFrequency)/2  "speed"
  BusCreator_DATA.c.cP.hFC.bVCHF.yawRate(PRESCAN_V2X_USER_CAM_yawRate)/1 -> BusCreator_DATA.c.cP.hFC.basicVehicleContainerHighFrequency(PRESCAN_V2X_USER_CAM_basicVehicleContainerHighFrequency)/9  "yawRate"
  BusCreator_DATA.c.cP.hFC.bVCHF.heading(PRESCAN_V2X_USER_CAM_heading)/1 -> BusCreator_DATA.c.cP.hFC.basicVehicleContainerHighFrequency(PRESCAN_V2X_USER_CAM_basicVehicleContainerHighFrequency)/1  "heading"
  BusCreator_DATA.c.cP.hFC.basicVehicleContainerHighFrequency(PRESCAN_V2X_USER_CAM_basicVehicleContainerHighFrequency)/1 -> BusCreator_DATA.c.cP.highFrequencyContainer(PRESCAN_V2X_USER_CAM_highFrequencyContainer)/1  "basicVehicleContainerHighFrequency"
  BusCreator_DATA.c.cP.basicContainer(PRESCAN_V2X_USER_CAM_basicContainer)/1 -> BusCreator_DATA.c.camParameters(PRESCAN_V2X_USER_CAM_camParameters)/1  "basicContainer"
  BusCreator_DATA.c.cP.highFrequencyContainer(PRESCAN_V2X_USER_CAM_highFrequencyContainer)/1 -> BusCreator_DATA.c.camParameters(PRESCAN_V2X_USER_CAM_camParameters)/2  "highFrequencyContainer"
  DATA.c.generationDeltaTime/1 -> BusCreator_DATA.cam(PRESCAN_V2X_USER_CAM_cam)/1  "generationDeltaTime"
  BusCreator_DATA.c.camParameters(PRESCAN_V2X_USER_CAM_camParameters)/1 -> BusCreator_DATA.cam(PRESCAN_V2X_USER_CAM_cam)/2  "camParameters"
  BusCreator_DATA.header(PRESCAN_V2X_USER_CAM_header)/1 -> BusCreator_DATA(PRESCAN_V2X_USER_CAM_DATA)/1  "header"
  BusCreator_DATA.cam(PRESCAN_V2X_USER_CAM_cam)/1 -> BusCreator_DATA(PRESCAN_V2X_USER_CAM_DATA)/2  "cam"
  BusCreator_HEADER(PRESCAN_HEADER)/1 -> BusCreator_PRESCAN_V2X_USER_CAM_MESSAGE(PRESCAN_V2X_USER_CAM_MESSAGE)/1  "HEADER"
  BusCreator_DATA(PRESCAN_V2X_USER_CAM_DATA)/1 -> BusCreator_PRESCAN_V2X_USER_CAM_MESSAGE(PRESCAN_V2X_USER_CAM_MESSAGE)/2  "DATA"
  BusCreator_PRESCAN_V2X_USER_CAM_MESSAGE(PRESCAN_V2X_USER_CAM_MESSAGE)/1 -> PRESCAN_V2X_USER_CAM_MESSAGE/1

== system v2x_cs/SteeringWheel_Pivot_Citroen_C3_Hatchback_1/Actuator ==
  Joint : Inport
  Bus Selector : BusSelector  OutputSignals=POSITION,ORIENTATION
  visu_Rotate : Subsystem  mask(RPYActuator){UniqueID=UniqueID, Object3DID=Rotate_ObjectID3D, TimeStep=TimeStep}
      mask prompts: UniqueID "Auto-Assigned: Unique ID"; Object3DID "Auto-Assigned: Child 3D Object ID"; TimeStep "Auto-Assigned: Upload Period [s]"
      mask help: Applies angles update to selected child object
      mask Help:
      | Applies position update to selected child object
      | 
      | - UniqueID (double)   : Unique ID of the parent actor
      | - Object3DID (string) : Name of the child 3D object
      mask Display: port_label('input', 1, ['visu_Rotate_' Object3DID])
  visu_Translate : Subsystem  mask(PositionActuator){UniqueID=UniqueID, Object3DID=Translate_ObjectID3D, TimeStep=TimeStep}
      mask prompts: UniqueID "Auto-Assigned: Unique ID"; Object3DID "Auto-Assigned: Child 3D Object ID"; TimeStep "Auto-Assigned: Upload Period [s]"
      mask help: Applies position update to selected child object
      mask Help:
      | Applies position update to selected child object
      | 
      | - UniqueID (double)   : Unique ID of the parent actor
      | - Object3DID (string) : Name of the child 3D object
      mask Display: port_label('input', 1, ['visu_Translate_' Object3DID])
  wires:
  Bus Selector/2 -> visu_Rotate/1(In1)  "<ORIENTATION>"
  Bus Selector/1 -> visu_Translate/1(In1)  "<POSITION>"
  Joint/1 -> Bus Selector/1

== system v2x_cs/SteeringWheel_pivot_Audi_A8_Sedan_1/Actuator ==
  Joint : Inport
  Bus Selector : BusSelector  OutputSignals=POSITION,ORIENTATION
  visu_Rotate : Subsystem  mask(RPYActuator){UniqueID=UniqueID, Object3DID=Rotate_ObjectID3D, TimeStep=TimeStep}
      mask prompts: UniqueID "Auto-Assigned: Unique ID"; Object3DID "Auto-Assigned: Child 3D Object ID"; TimeStep "Auto-Assigned: Upload Period [s]"
      mask help: Applies angles update to selected child object
      mask Help:
      | Applies position update to selected child object
      | 
      | - UniqueID (double)   : Unique ID of the parent actor
      | - Object3DID (string) : Name of the child 3D object
      mask Display: port_label('input', 1, ['visu_Rotate_' Object3DID])
  visu_Translate : Subsystem  mask(PositionActuator){UniqueID=UniqueID, Object3DID=Translate_ObjectID3D, TimeStep=TimeStep}
      mask prompts: UniqueID "Auto-Assigned: Unique ID"; Object3DID "Auto-Assigned: Child 3D Object ID"; TimeStep "Auto-Assigned: Upload Period [s]"
      mask help: Applies position update to selected child object
      mask Help:
      | Applies position update to selected child object
      | 
      | - UniqueID (double)   : Unique ID of the parent actor
      | - Object3DID (string) : Name of the child 3D object
      mask Display: port_label('input', 1, ['visu_Translate_' Object3DID])
  wires:
  Bus Selector/2 -> visu_Rotate/1(In1)  "<ORIENTATION>"
  Bus Selector/1 -> visu_Translate/1(In1)  "<POSITION>"
  Joint/1 -> Bus Selector/1

== system v2x_cs/SteeringWheel_pivot_BMW_X5_SUV_1/Actuator ==
  Joint : Inport
  Bus Selector : BusSelector  OutputSignals=POSITION,ORIENTATION
  visu_Rotate : Subsystem  mask(RPYActuator){UniqueID=UniqueID, Object3DID=Rotate_ObjectID3D, TimeStep=TimeStep}
      mask prompts: UniqueID "Auto-Assigned: Unique ID"; Object3DID "Auto-Assigned: Child 3D Object ID"; TimeStep "Auto-Assigned: Upload Period [s]"
      mask help: Applies angles update to selected child object
      mask Help:
      | Applies position update to selected child object
      | 
      | - UniqueID (double)   : Unique ID of the parent actor
      | - Object3DID (string) : Name of the child 3D object
      mask Display: port_label('input', 1, ['visu_Rotate_' Object3DID])
  visu_Translate : Subsystem  mask(PositionActuator){UniqueID=UniqueID, Object3DID=Translate_ObjectID3D, TimeStep=TimeStep}
      mask prompts: UniqueID "Auto-Assigned: Unique ID"; Object3DID "Auto-Assigned: Child 3D Object ID"; TimeStep "Auto-Assigned: Upload Period [s]"
      mask help: Applies position update to selected child object
      mask Help:
      | Applies position update to selected child object
      | 
      | - UniqueID (double)   : Unique ID of the parent actor
      | - Object3DID (string) : Name of the child 3D object
      mask Display: port_label('input', 1, ['visu_Translate_' Object3DID])
  wires:
  Bus Selector/2 -> visu_Rotate/1(In1)  "<ORIENTATION>"
  Bus Selector/1 -> visu_Translate/1(In1)  "<POSITION>"
  Joint/1 -> Bus Selector/1

== system v2x_cs/SteeringWheel_pivot_BMW_Z3_Convertible_1/Actuator ==
  Joint : Inport
  Bus Selector : BusSelector  OutputSignals=POSITION,ORIENTATION
  visu_Rotate : Subsystem  mask(RPYActuator){UniqueID=UniqueID, Object3DID=Rotate_ObjectID3D, TimeStep=TimeStep}
      mask prompts: UniqueID "Auto-Assigned: Unique ID"; Object3DID "Auto-Assigned: Child 3D Object ID"; TimeStep "Auto-Assigned: Upload Period [s]"
      mask help: Applies angles update to selected child object
      mask Help:
      | Applies position update to selected child object
      | 
      | - UniqueID (double)   : Unique ID of the parent actor
      | - Object3DID (string) : Name of the child 3D object
      mask Display: port_label('input', 1, ['visu_Rotate_' Object3DID])
  visu_Translate : Subsystem  mask(PositionActuator){UniqueID=UniqueID, Object3DID=Translate_ObjectID3D, TimeStep=TimeStep}
      mask prompts: UniqueID "Auto-Assigned: Unique ID"; Object3DID "Auto-Assigned: Child 3D Object ID"; TimeStep "Auto-Assigned: Upload Period [s]"
      mask help: Applies position update to selected child object
      mask Help:
      | Applies position update to selected child object
      | 
      | - UniqueID (double)   : Unique ID of the parent actor
      | - Object3DID (string) : Name of the child 3D object
      mask Display: port_label('input', 1, ['visu_Translate_' Object3DID])
  wires:
  Bus Selector/2 -> visu_Rotate/1(In1)  "<ORIENTATION>"
  Bus Selector/1 -> visu_Translate/1(In1)  "<POSITION>"
  Joint/1 -> Bus Selector/1

== system v2x_cs/SteeringWheel_pivot_Mazda_RX8_Coupe_1/Actuator ==
  Joint : Inport
  Bus Selector : BusSelector  OutputSignals=POSITION,ORIENTATION
  visu_Rotate : Subsystem  mask(RPYActuator){UniqueID=UniqueID, Object3DID=Rotate_ObjectID3D, TimeStep=TimeStep}
      mask prompts: UniqueID "Auto-Assigned: Unique ID"; Object3DID "Auto-Assigned: Child 3D Object ID"; TimeStep "Auto-Assigned: Upload Period [s]"
      mask help: Applies angles update to selected child object
      mask Help:
      | Applies position update to selected child object
      | 
      | - UniqueID (double)   : Unique ID of the parent actor
      | - Object3DID (string) : Name of the child 3D object
      mask Display: port_label('input', 1, ['visu_Rotate_' Object3DID])
  visu_Translate : Subsystem  mask(PositionActuator){UniqueID=UniqueID, Object3DID=Translate_ObjectID3D, TimeStep=TimeStep}
      mask prompts: UniqueID "Auto-Assigned: Unique ID"; Object3DID "Auto-Assigned: Child 3D Object ID"; TimeStep "Auto-Assigned: Upload Period [s]"
      mask help: Applies position update to selected child object
      mask Help:
      | Applies position update to selected child object
      | 
      | - UniqueID (double)   : Unique ID of the parent actor
      | - Object3DID (string) : Name of the child 3D object
      mask Display: port_label('input', 1, ['visu_Translate_' Object3DID])
  wires:
  Bus Selector/2 -> visu_Rotate/1(In1)  "<ORIENTATION>"
  Bus Selector/1 -> visu_Translate/1(In1)  "<POSITION>"
  Joint/1 -> Bus Selector/1

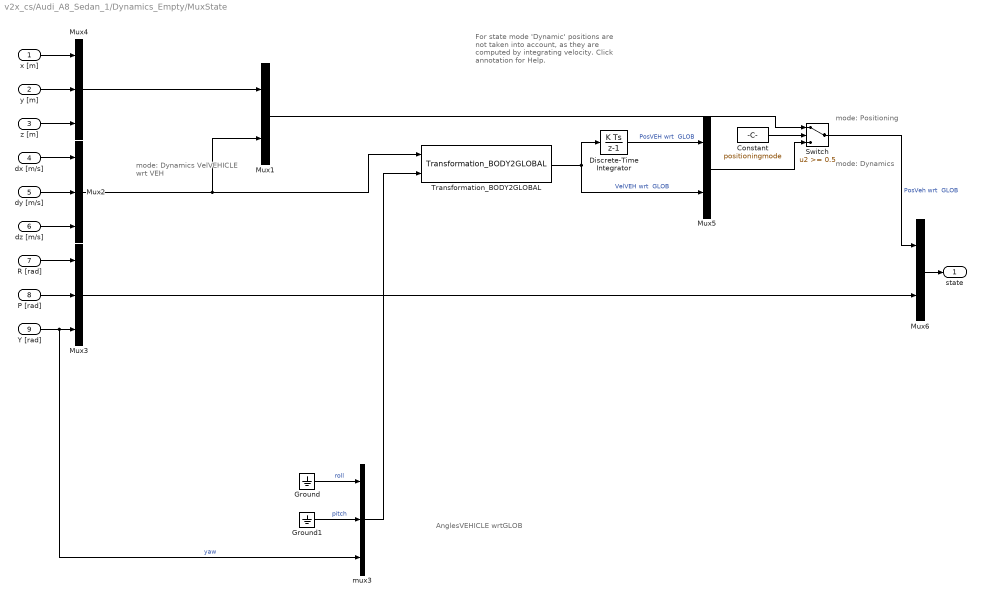
== system v2x_cs/Audi_A8_Sedan_1/Dynamics_Empty/MuxState ==
  note: mode: Dynamics
  note: mode: Positioning
  note: mode: Dynamics
      | VelVEHICLE
      | wrt VEH
  note: AnglesVEHICLE
      | wrtGLOB
  note: For state mode 'Dynamic' positions
      | are not taken into account, as they
      | are computed by integrating velocity.
      | Click annotation for Help.
  x [m] : Inport  SampleTime=TimeStep
  y [m] : Inport  Port=2  SampleTime=TimeStep
  z [m] : Inport  Port=3  SampleTime=TimeStep
  dx [m/s] : Inport  Port=4  SampleTime=TimeStep
  dy [m/s] : Inport  Port=5  SampleTime=TimeStep
  dz [m/s] : Inport  Port=6  SampleTime=TimeStep
  R [rad] : Inport  Port=7  SampleTime=TimeStep
  P [rad] : Inport  Port=8  SampleTime=TimeStep
  Y [rad] : Inport  Port=9  SampleTime=TimeStep
  Constant : Constant  DisableCoverage=on  Value=positioningmode
  Discrete-Time Integrator : DiscreteIntegrator  SampleTime=TimeStep  ICPrevOutput=DiscIntNeverNeededParam  ICPrevScaledInput=DiscIntNeverNeededParam
  Ground : Ground
  Ground1 : Ground
  Mux1 : Mux  Inputs=[3 3]
  Mux2 : Mux  Inputs=3
  Mux3 : Mux  Inputs=3
  Mux4 : Mux  Inputs=3
  Mux5 : Mux  Inputs=[3 3]
  Mux6 : Mux  Inputs=[6 3]
  Switch : Switch  Threshold=0.5
  Transformation_BODY2GLOBAL : PreScanSimulinkLibrary/Simple_Vehicle_Dynamics/Chassis/MuxDynState/Transformation_BODY2GLOBAL  SystemSampleTime=-1
  mux3 : Mux  Inputs=3
  state : Outport
  wires:
  Constant/1 -> Switch/2
  Mux6/1 -> state/1
  Mux4/1 -> Mux1/1
  Mux5/1 -> Switch/3
  Mux1/1 -> Switch/1
  Switch/1 -> Mux6/1  "PosVeh wrt  GLOB"
  P [rad]/1 -> Mux3/2
  R [rad]/1 -> Mux3/1
  dz [m/s]/1 -> Mux2/3
  dy [m/s]/1 -> Mux2/2
  dx [m/s]/1 -> Mux2/1
  z [m]/1 -> Mux4/3
  y [m]/1 -> Mux4/2
  x [m]/1 -> Mux4/1
  Ground1/1 -> mux3/2  "pitch"
  Y [rad]/1 -> mux3/3, Mux3/3  "yaw"
  Mux3/1 -> Mux6/2
  Transformation_BODY2GLOBAL/1 -> Discrete-Time Integrator/1, Mux5/2  "VelVEH wrt  GLOB"
  mux3/1 -> Transformation_BODY2GLOBAL/2
  Ground/1 -> mux3/1  "roll"
  Mux2/1 -> Mux1/2, Transformation_BODY2GLOBAL/1
  Discrete-Time Integrator/1 -> Mux5/1  "PosVEH wrt  GLOB"

== system v2x_cs/Audi_A8_Sedan_1/SELF_Demux/compas converter ==
  rotz [rad] : Inport
  cart2compas : Subsystem
  rad2deg : Gain  Gain=180/pi
  heading [deg] : Outport
  wires:
  rad2deg/1 -> cart2compas/1(Angle [deg])
  rotz [rad]/1 -> rad2deg/1
  cart2compas/1(heading [deg]) -> heading [deg]/1

== system v2x_cs/Audi_A8_Sedan_1/V2X_29_CAM_Filter/Filter ==
  In : Inport
  Filter : MATLAB Function  TreatAsAtomicUnit=on
  Zero : Constant  Value=0  OutDataTypeStr=Bus: PRESCAN_V2X_USER_CAM_MESSAGE
  Out : Outport
  wires:
  Zero/1 -> Filter/2(z)
  Filter/1(y) -> Out/1
  In/1 -> Filter/1(u)

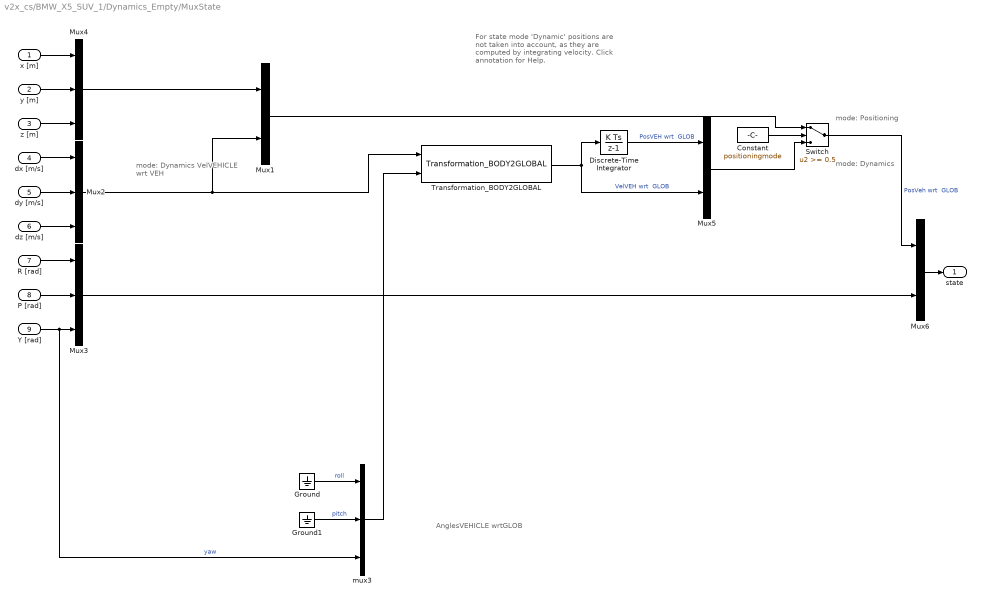
== system v2x_cs/BMW_X5_SUV_1/Dynamics_Empty/MuxState ==
  note: mode: Dynamics
  note: mode: Positioning
  note: mode: Dynamics
      | VelVEHICLE
      | wrt VEH
  note: AnglesVEHICLE
      | wrtGLOB
  note: For state mode 'Dynamic' positions
      | are not taken into account, as they
      | are computed by integrating velocity.
      | Click annotation for Help.
  x [m] : Inport  SampleTime=TimeStep
  y [m] : Inport  Port=2  SampleTime=TimeStep
  z [m] : Inport  Port=3  SampleTime=TimeStep
  dx [m/s] : Inport  Port=4  SampleTime=TimeStep
  dy [m/s] : Inport  Port=5  SampleTime=TimeStep
  dz [m/s] : Inport  Port=6  SampleTime=TimeStep
  R [rad] : Inport  Port=7  SampleTime=TimeStep
  P [rad] : Inport  Port=8  SampleTime=TimeStep
  Y [rad] : Inport  Port=9  SampleTime=TimeStep
  Constant : Constant  DisableCoverage=on  Value=positioningmode
  Discrete-Time Integrator : DiscreteIntegrator  SampleTime=TimeStep  ICPrevOutput=DiscIntNeverNeededParam  ICPrevScaledInput=DiscIntNeverNeededParam
  Ground : Ground
  Ground1 : Ground
  Mux1 : Mux  Inputs=[3 3]
  Mux2 : Mux  Inputs=3
  Mux3 : Mux  Inputs=3
  Mux4 : Mux  Inputs=3
  Mux5 : Mux  Inputs=[3 3]
  Mux6 : Mux  Inputs=[6 3]
  Switch : Switch  Threshold=0.5
  Transformation_BODY2GLOBAL : PreScanSimulinkLibrary/Simple_Vehicle_Dynamics/Chassis/MuxDynState/Transformation_BODY2GLOBAL  SystemSampleTime=-1
  mux3 : Mux  Inputs=3
  state : Outport
  wires:
  Constant/1 -> Switch/2
  Mux6/1 -> state/1
  Mux4/1 -> Mux1/1
  Mux5/1 -> Switch/3
  Mux1/1 -> Switch/1
  Switch/1 -> Mux6/1  "PosVeh wrt  GLOB"
  P [rad]/1 -> Mux3/2
  R [rad]/1 -> Mux3/1
  dz [m/s]/1 -> Mux2/3
  dy [m/s]/1 -> Mux2/2
  dx [m/s]/1 -> Mux2/1
  z [m]/1 -> Mux4/3
  y [m]/1 -> Mux4/2
  x [m]/1 -> Mux4/1
  Ground1/1 -> mux3/2  "pitch"
  Y [rad]/1 -> mux3/3, Mux3/3  "yaw"
  Mux3/1 -> Mux6/2
  Transformation_BODY2GLOBAL/1 -> Discrete-Time Integrator/1, Mux5/2  "VelVEH wrt  GLOB"
  mux3/1 -> Transformation_BODY2GLOBAL/2
  Ground/1 -> mux3/1  "roll"
  Mux2/1 -> Mux1/2, Transformation_BODY2GLOBAL/1
  Discrete-Time Integrator/1 -> Mux5/1  "PosVEH wrt  GLOB"

== system v2x_cs/BMW_X5_SUV_1/SELF_Demux/compas converter ==
  rotz [rad] : Inport
  cart2compas : Subsystem
  rad2deg : Gain  Gain=180/pi
  heading [deg] : Outport
  wires:
  rad2deg/1 -> cart2compas/1(Angle [deg])
  rotz [rad]/1 -> rad2deg/1
  cart2compas/1(heading [deg]) -> heading [deg]/1

== system v2x_cs/BMW_X5_SUV_1/V2X_30_CAM_Filter/Filter ==
  In : Inport
  Filter : MATLAB Function  TreatAsAtomicUnit=on
  Zero : Constant  Value=0  OutDataTypeStr=Bus: PRESCAN_V2X_USER_CAM_MESSAGE
  Out : Outport
  wires:
  Zero/1 -> Filter/2(z)
  Filter/1(y) -> Out/1
  In/1 -> Filter/1(u)

== system v2x_cs/BMW_Z3_Convertible_1/Dynamics_Empty/MuxState ==
  note: mode: Dynamics
  note: mode: Positioning
  note: mode: Dynamics
      | VelVEHICLE
      | wrt VEH
  note: AnglesVEHICLE
      | wrtGLOB
  note: For state mode 'Dynamic' positions
      | are not taken into account, as they
      | are computed by integrating velocity.
      | Click annotation for Help.
  x [m] : Inport  SampleTime=TimeStep
  y [m] : Inport  Port=2  SampleTime=TimeStep
  z [m] : Inport  Port=3  SampleTime=TimeStep
  dx [m/s] : Inport  Port=4  SampleTime=TimeStep
  dy [m/s] : Inport  Port=5  SampleTime=TimeStep
  dz [m/s] : Inport  Port=6  SampleTime=TimeStep
  R [rad] : Inport  Port=7  SampleTime=TimeStep
  P [rad] : Inport  Port=8  SampleTime=TimeStep
  Y [rad] : Inport  Port=9  SampleTime=TimeStep
  Constant : Constant  DisableCoverage=on  Value=positioningmode
  Discrete-Time Integrator : DiscreteIntegrator  SampleTime=TimeStep  ICPrevOutput=DiscIntNeverNeededParam  ICPrevScaledInput=DiscIntNeverNeededParam
  Ground : Ground
  Ground1 : Ground
  Mux1 : Mux  Inputs=[3 3]
  Mux2 : Mux  Inputs=3
  Mux3 : Mux  Inputs=3
  Mux4 : Mux  Inputs=3
  Mux5 : Mux  Inputs=[3 3]
  Mux6 : Mux  Inputs=[6 3]
  Switch : Switch  Threshold=0.5
  Transformation_BODY2GLOBAL : PreScanSimulinkLibrary/Simple_Vehicle_Dynamics/Chassis/MuxDynState/Transformation_BODY2GLOBAL  SystemSampleTime=-1
  mux3 : Mux  Inputs=3
  state : Outport
  wires:
  Constant/1 -> Switch/2
  Mux6/1 -> state/1
  Mux4/1 -> Mux1/1
  Mux5/1 -> Switch/3
  Mux1/1 -> Switch/1
  Switch/1 -> Mux6/1  "PosVeh wrt  GLOB"
  P [rad]/1 -> Mux3/2
  R [rad]/1 -> Mux3/1
  dz [m/s]/1 -> Mux2/3
  dy [m/s]/1 -> Mux2/2
  dx [m/s]/1 -> Mux2/1
  z [m]/1 -> Mux4/3
  y [m]/1 -> Mux4/2
  x [m]/1 -> Mux4/1
  Ground1/1 -> mux3/2  "pitch"
  Y [rad]/1 -> mux3/3, Mux3/3  "yaw"
  Mux3/1 -> Mux6/2
  Transformation_BODY2GLOBAL/1 -> Discrete-Time Integrator/1, Mux5/2  "VelVEH wrt  GLOB"
  mux3/1 -> Transformation_BODY2GLOBAL/2
  Ground/1 -> mux3/1  "roll"
  Mux2/1 -> Mux1/2, Transformation_BODY2GLOBAL/1
  Discrete-Time Integrator/1 -> Mux5/1  "PosVEH wrt  GLOB"

== system v2x_cs/BMW_Z3_Convertible_1/SELF_Demux/compas converter ==
  rotz [rad] : Inport
  cart2compas : Subsystem
  rad2deg : Gain  Gain=180/pi
  heading [deg] : Outport
  wires:
  rad2deg/1 -> cart2compas/1(Angle [deg])
  rotz [rad]/1 -> rad2deg/1
  cart2compas/1(heading [deg]) -> heading [deg]/1

== system v2x_cs/BMW_Z3_Convertible_1/V2X_28_CAM_Filter/Filter ==
  In : Inport
  Filter : MATLAB Function  TreatAsAtomicUnit=on
  Zero : Constant  Value=0  OutDataTypeStr=Bus: PRESCAN_V2X_USER_CAM_MESSAGE
  Out : Outport
  wires:
  Zero/1 -> Filter/2(z)
  Filter/1(y) -> Out/1
  In/1 -> Filter/1(u)

== system v2x_cs/Citroen_C3_Hatchback_1/Dynamics_Empty/MuxState ==
  note: mode: Dynamics
  note: mode: Positioning
  note: mode: Dynamics
      | VelVEHICLE
      | wrt VEH
  note: AnglesVEHICLE
      | wrtGLOB
  note: For state mode 'Dynamic' positions
      | are not taken into account, as they
      | are computed by integrating velocity.
      | Click annotation for Help.
  x [m] : Inport  SampleTime=TimeStep
  y [m] : Inport  Port=2  SampleTime=TimeStep
  z [m] : Inport  Port=3  SampleTime=TimeStep
  dx [m/s] : Inport  Port=4  SampleTime=TimeStep
  dy [m/s] : Inport  Port=5  SampleTime=TimeStep
  dz [m/s] : Inport  Port=6  SampleTime=TimeStep
  R [rad] : Inport  Port=7  SampleTime=TimeStep
  P [rad] : Inport  Port=8  SampleTime=TimeStep
  Y [rad] : Inport  Port=9  SampleTime=TimeStep
  Constant : Constant  DisableCoverage=on  Value=positioningmode
  Discrete-Time Integrator : DiscreteIntegrator  SampleTime=TimeStep  ICPrevOutput=DiscIntNeverNeededParam  ICPrevScaledInput=DiscIntNeverNeededParam
  Ground : Ground
  Ground1 : Ground
  Mux1 : Mux  Inputs=[3 3]
  Mux2 : Mux  Inputs=3
  Mux3 : Mux  Inputs=3
  Mux4 : Mux  Inputs=3
  Mux5 : Mux  Inputs=[3 3]
  Mux6 : Mux  Inputs=[6 3]
  Switch : Switch  Threshold=0.5
  Transformation_BODY2GLOBAL : PreScanSimulinkLibrary/Simple_Vehicle_Dynamics/Chassis/MuxDynState/Transformation_BODY2GLOBAL  SystemSampleTime=-1
  mux3 : Mux  Inputs=3
  state : Outport
  wires:
  Constant/1 -> Switch/2
  Mux6/1 -> state/1
  Mux4/1 -> Mux1/1
  Mux5/1 -> Switch/3
  Mux1/1 -> Switch/1
  Switch/1 -> Mux6/1  "PosVeh wrt  GLOB"
  P [rad]/1 -> Mux3/2
  R [rad]/1 -> Mux3/1
  dz [m/s]/1 -> Mux2/3
  dy [m/s]/1 -> Mux2/2
  dx [m/s]/1 -> Mux2/1
  z [m]/1 -> Mux4/3
  y [m]/1 -> Mux4/2
  x [m]/1 -> Mux4/1
  Ground1/1 -> mux3/2  "pitch"
  Y [rad]/1 -> mux3/3, Mux3/3  "yaw"
  Mux3/1 -> Mux6/2
  Transformation_BODY2GLOBAL/1 -> Discrete-Time Integrator/1, Mux5/2  "VelVEH wrt  GLOB"
  mux3/1 -> Transformation_BODY2GLOBAL/2
  Ground/1 -> mux3/1  "roll"
  Mux2/1 -> Mux1/2, Transformation_BODY2GLOBAL/1
  Discrete-Time Integrator/1 -> Mux5/1  "PosVEH wrt  GLOB"

== system v2x_cs/Citroen_C3_Hatchback_1/SELF_Demux/compas converter ==
  rotz [rad] : Inport
  cart2compas : Subsystem
  rad2deg : Gain  Gain=180/pi
  heading [deg] : Outport
  wires:
  rad2deg/1 -> cart2compas/1(Angle [deg])
  rotz [rad]/1 -> rad2deg/1
  cart2compas/1(heading [deg]) -> heading [deg]/1

== system v2x_cs/Citroen_C3_Hatchback_1/V2X_31_CAM_Filter/Filter ==
  In : Inport
  Filter : MATLAB Function  TreatAsAtomicUnit=on
  Zero : Constant  Value=0  OutDataTypeStr=Bus: PRESCAN_V2X_USER_CAM_MESSAGE
  Out : Outport
  wires:
  Zero/1 -> Filter/2(z)
  Filter/1(y) -> Out/1
  In/1 -> Filter/1(u)
